simulink model "CO2_Storage_Room"  (R2022b)
settings: Solver=FixedStepAuto  StartTime=0.0  StopTime=20000  FixedStep=1  RelTol=1e-3
model workspace (MAT data in the model file):
  P0 = 100
  T0 = 500
  m0 = 320000
settings Model: Creator=Crapon  LastModifiedBy=Crapon

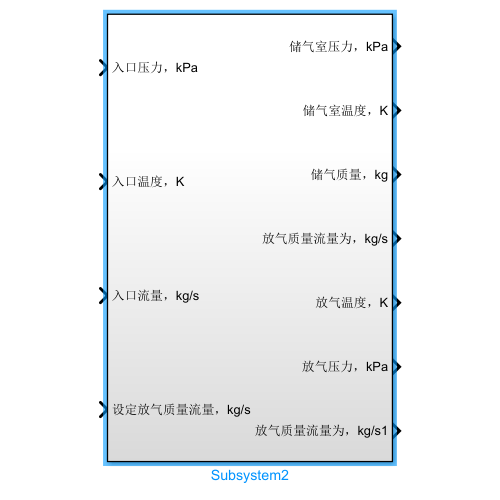
[thumbnail: Simulink's stored preview of the top-level diagram]
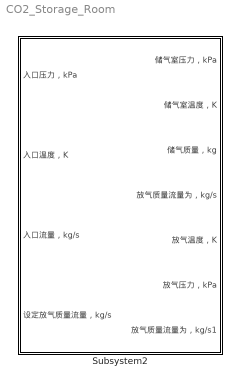
== system CO2_Storage_Room ==
  Subsystem2 : Subsystem

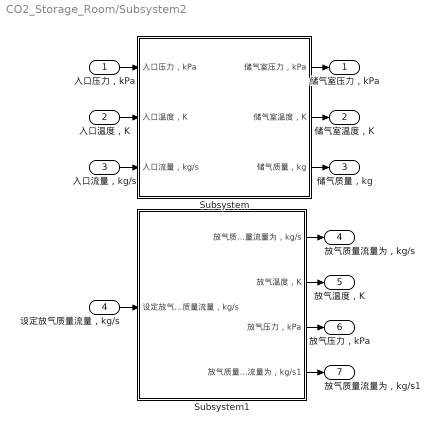
== system CO2_Storage_Room/Subsystem2 ==
  入口压力，kPa : Inport
  入口温度，K : Inport  Port=2
  入口流量，kg/s : Inport  Port=3
  设定放气质量流量，kg/s : Inport  Port=4
  Subsystem : Subsystem
  Subsystem1 : Subsystem
  储气室压力，kPa : Outport
  储气室温度，K : Outport  Port=2
  储气质量，kg : Outport  Port=3
  放气质量流量为，kg/s : Outport  Port=4
  放气温度，K : Outport  Port=5
  放气压力，kPa : Outport  Port=6
  放气质量流量为，kg/s1 : Outport  Port=7
  wires:
  Subsystem1/3(放气压力，kPa) -> 放气压力，kPa/1
  Subsystem1/4(放气质量流量为，kg/s1) -> 放气质量流量为，kg/s1/1
  入口压力，kPa/1 -> Subsystem/1(入口压力，kPa)
  入口温度，K/1 -> Subsystem/2(入口温度，K)
  Subsystem/2(储气室温度，K) -> 储气室温度，K/1
  入口流量，kg/s/1 -> Subsystem/3(入口流量，kg/s)
  Subsystem/1(储气室压力，kPa) -> 储气室压力，kPa/1
  Subsystem/3(储气质量，kg) -> 储气质量，kg/1
  设定放气质量流量，kg/s/1 -> Subsystem1/1(设定放气质量流量，kg/s)
  Subsystem1/2(放气温度，K) -> 放气温度，K/1
  Subsystem1/1(放气质量流量为，kg/s) -> 放气质量流量为，kg/s/1

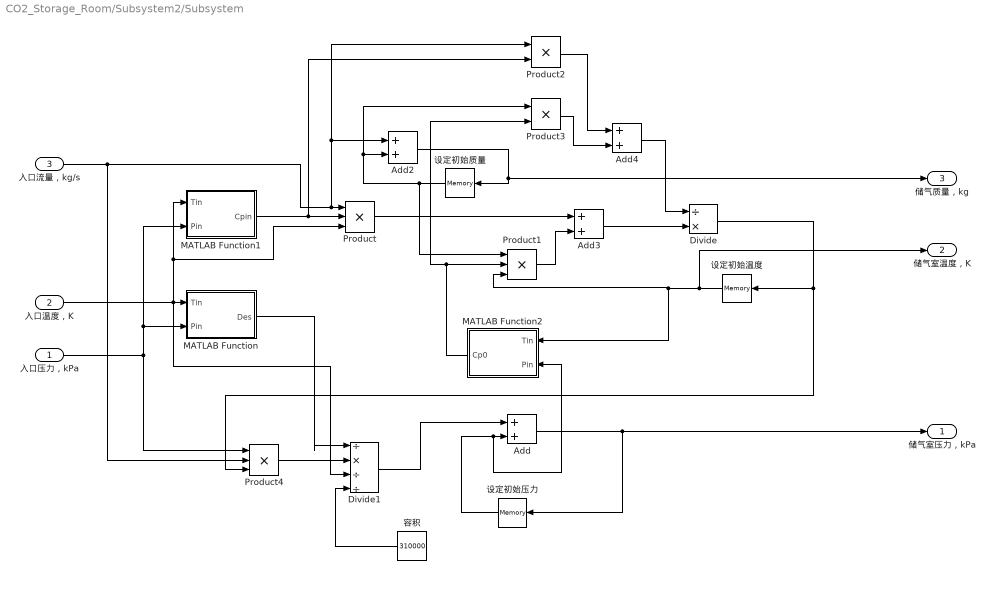
== system CO2_Storage_Room/Subsystem2/Subsystem ==
  入口压力，kPa : Inport
  入口温度，K : Inport  Port=2
  入口流量，kg/s : Inport  Port=3
  Add{,2..4} (4 alike) : Sum
  Divide : Product  Inputs=/*
  Divide1 : Product  Inputs=/*//
  MATLAB Function : MATLAB Function  TreatAsAtomicUnit=on
  MATLAB Function1 : MATLAB Function  TreatAsAtomicUnit=on
  MATLAB Function2 : MATLAB Function  TreatAsAtomicUnit=on
  Product : Product  Inputs=3
  Product1 : Product  Inputs=3
  Product2 : Product
  Product3 : Product
  Product4 : Product  Inputs=3
  容积 : Constant  Value=310000
  设定初始压力 : Memory  InitialCondition=P0
  设定初始温度 : Memory  InitialCondition=T0
  设定初始质量 : Memory  InitialCondition=m0
  储气室压力，kPa : Outport
  储气室温度，K : Outport  Port=2
  储气质量，kg : Outport  Port=3
  wires:
  入口流量，kg/s/1 -> Product4/2, Product2/1, Add2/1, Product/1
  设定初始质量/1 -> Product1/1, Product3/1, Add2/2
  Product2/1 -> Add4/1
  MATLAB Function1/1(Cpin) -> Product/2, Product2/2
  Product4/1 -> Divide1/2
  MATLAB Function2/1(Cp0) -> Product1/2, Product3/2
  Divide1/1 -> Add/1
  入口温度，K/1 -> MATLAB Function1/1(Tin), Product/3, MATLAB Function/1(Tin), Divide1/3
  Product1/1 -> Add3/2
  Add/1 -> 储气室压力，kPa/1, 设定初始压力/1
  入口压力，kPa/1 -> Product4/1, MATLAB Function1/2(Pin), MATLAB Function/2(Pin)
  Add4/1 -> Divide/1
  设定初始压力/1 -> MATLAB Function2/2(Pin), Add/2
  容积/1 -> Divide1/4
  Product3/1 -> Add4/2
  MATLAB Function/1(Des) -> Divide1/1
  Add3/1 -> Divide/2
  Product/1 -> Add3/1
  Divide/1 -> Product4/3, 设定初始温度/1
  Add2/1 -> 设定初始质量/1, 储气质量，kg/1
  设定初始温度/1 -> 储气室温度，K/1, MATLAB Function2/1(Tin), Product1/3

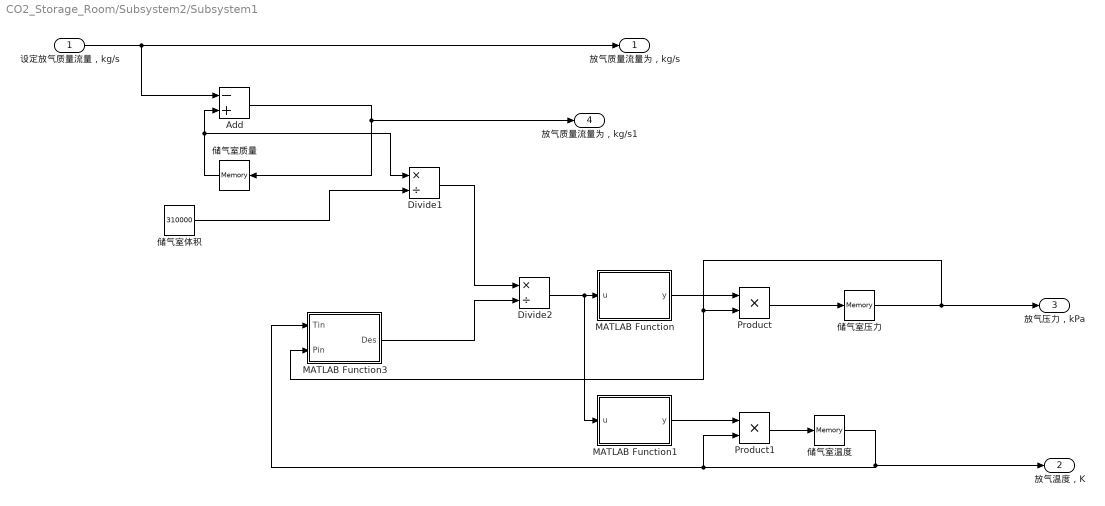
== system CO2_Storage_Room/Subsystem2/Subsystem1 ==
  设定放气质量流量，kg/s : Inport
  Add : Sum  Inputs=-+
  Divide1 : Product  Inputs=*/
  Divide2 : Product  Inputs=*/
  MATLAB Function : MATLAB Function  TreatAsAtomicUnit=on
  MATLAB Function1 : MATLAB Function  TreatAsAtomicUnit=on
  MATLAB Function3 : MATLAB Function  TreatAsAtomicUnit=on
  Product : Product
  Product1 : Product
  储气室体积 : Constant  Value=310000
  储气室压力 : Memory  InitialCondition=P0
  储气室温度 : Memory  InitialCondition=T0
  储气室质量 : Memory  InitialCondition=m0
  放气质量流量为，kg/s : Outport
  放气温度，K : Outport  Port=2
  放气压力，kPa : Outport  Port=3
  放气质量流量为，kg/s1 : Outport  Port=4
  wires:
  设定放气质量流量，kg/s/1 -> 放气质量流量为，kg/s/1, Add/1
  MATLAB Function3/1(Des) -> Divide2/2
  储气室质量/1 -> Divide1/1, Add/2
  Add/1 -> 放气质量流量为，kg/s1/1, 储气室质量/1
  储气室体积/1 -> Divide1/2
  Divide1/1 -> Divide2/1
  Divide2/1 -> MATLAB Function1/1(u), MATLAB Function/1(u)
  储气室压力/1 -> Product/2, MATLAB Function3/2(Pin), 放气压力，kPa/1
  Product/1 -> 储气室压力/1
  MATLAB Function1/1(y) -> Product1/1
  Product1/1 -> 储气室温度/1
  储气室温度/1 -> MATLAB Function3/1(Tin), Product1/2, 放气温度，K/1
  MATLAB Function/1(y) -> Product/1

== matlab function CO2_Storage_Room/Subsystem2/Subsystem/MATLAB Function ==
  data: Tin input; Des output; Pin input
function Des = fcn(Tin,Pin)
coder.extrinsic('refpropm');
Des=zeros(1);
Des = refpropm('D','T',Tin,'P',Pin,'CO2');

== matlab function CO2_Storage_Room/Subsystem2/Subsystem/MATLAB Function2 ==
  data: Tin input; Cp0 output; Pin input
function Cp0 = fcn(Tin,Pin)
coder.extrinsic('refpropm');
Cp0=zeros(1);
Cp0 = refpropm('C','T',Tin,'P',Pin,'CO2');

== matlab function CO2_Storage_Room/Subsystem2/Subsystem1/MATLAB Function ==
  data: u input; y output
function y = fcn(u)

y = u^1.295;

== matlab function CO2_Storage_Room/Subsystem2/Subsystem1/MATLAB Function3 ==
  data: Tin input; Des output; Pin input
function Des = fcn(Tin,Pin)
coder.extrinsic('refpropm');
Des=zeros(1);
Des = refpropm('D','T',Tin,'P',Pin,'CO2');

== matlab function CO2_Storage_Room/Subsystem2/Subsystem1/MATLAB Function1 ==
  data: u input; y output
function y = fcn(u)

y = u^0.295;

== matlab function CO2_Storage_Room/Subsystem2/Subsystem/MATLAB Function1 ==
  data: Tin input; Cpin output; Pin input
function Cpin = fcn(Tin,Pin)
coder.extrinsic('refpropm');
Cpin=zeros(1);
Cpin = refpropm('C','T',Tin,'P',Pin,'CO2');
